simulink model "sim_all"  (R2020a)
settings: Solver=VariableStepAuto  StartTime=0.0  StopTime=2000  RelTol=1e-3
values from neighbouring files (symbols this model uses):
  a1 = rho * D^4 * alpha1    (= 0.000388302366464)    [data_current.m]
  a2 = -rho * D^3 * alpha2 * (1 - omega)    (= 0.0037030698432)    [data_current.m]
  alpha1 = 0.0113    [data_current.m]
  alpha2 = -0.0091    [data_current.m]
  cornerA = [43.781381 ... (first row only)    [missionC.m]
  cornerB = [43.780975 ... (first row only)    [missionC.m]
  cornerC = [43.780189 ... (first row only)    [missionC.m]
  cornerD = [43.780602 ... (first row only)    [missionC.m]
  ctrl_clockwise = false    [controller.m]
  ctrl_int_bound_or = 0.1    [controller.m]
  ctrl_int_bound_pos = 1    [controller.m]
  ctrl_k_or = 1    [controller.m]
  ctrl_k_pos = 1/3    (= 0.333333333333)    [controller.m]
  ctrl_Ki_vel = 100    [controller.m]
  ctrl_Kp_v_pos = 200    [controller.m]
  ctrl_Kp_vel = 200    [controller.m]
  ctrl_TAM = [  1     1           0           0               0       0;               0     0           1           1               0       0;               0     0           0           0               1       1;               0     0  -(ctrl_r+ctrl_dc)  ctrl_r+ctrl_dc    0       0;               0     0           0           0            -ctrl_r    ctrl_r;           -ctrl_r ctrl_r        0           0       ...(+19 chars)    [controller.m]
  ctrl_Ts = 0.1    [controller.m]
  ctrl_va_uncontrolled = 0.15    [controller.m]
  ctrl_vel_uncontrolled = 0.5    [controller.m]
  D = 0.076    [data_current.m]
  dead_zone_limit = 31.5    [data_current.m]
  depth = 5    [missionC.m]
  distanceFromWall = 8    [missionC.m]
  initInspectedSide = 2    [missionC.m]
  initPoint = [ 43.780796 ... (first row only)    [missionC.m]
  mod_A = pi*mod_R*mod_R    [model.m]
  mod_Cd_F = 0.45    [model.m]
  mod_Cd_M = 0.4    [model.m]
  mod_eta_init = [mod_xNorth; mod_yEast; -mod_zDown; 0; 0; 0]    [model.m]
  mod_g = 9.81    [model.m]
  mod_h0 = 0    [model.m]
  mod_Ixx = mod_Io(1,1)    [model.m]
  mod_Iyy = mod_Io(2,2)    [model.m]
  mod_Izz = mod_Io(3,3)    [model.m]
  mod_Kp_dot = 0    [model.m]
  mod_lat0 = 43.780189    [model.m]
  mod_lon0 = 11.282698    [model.m]
  mod_m = 100    [model.m]
  mod_Mq_dot = mod_Kp_dot    (= 0)    [model.m]
  mod_ni_init = [0; 0; 0; 0; 0; 0]    [model.m]
  mod_Nr_dot = mod_Kp_dot    (= 0)    [model.m]
  mod_p1 = [0; mod_R; 0]    [model.m]
  mod_p2 = [0; -mod_R; 0]    [model.m]
  mod_p3 = [0; 0; (mod_R + mod_z_cm)]    [model.m]
  mod_p4 = [0; 0; -(mod_R + mod_z_cm)]    [model.m]
  mod_p5 = [mod_R; 0; 0]    [model.m]
  mod_p6 = [-mod_R; 0; 0]    [model.m]
  mod_R = ((3*mod_Vol)/(4*pi))^(1/3)    [model.m]
  mod_Rm = (4*mod_R)/(3*pi)    [model.m]
  mod_t1 = [1; 0; 0]    [model.m]
  mod_t2 = [1; 0; 0]    [model.m]
  mod_t3 = [0; 1; 0]    [model.m]
  mod_t4 = [0; 1; 0]    [model.m]
  mod_t5 = [0; 0; 1]    [model.m]
  mod_t6 = [0; 0; 1]    [model.m]
  mod_W = mod_m*mod_g    (= 981)    [model.m]
  mod_Xu_dot = (2/3)*mod_rho_AUV*pi*(mod_R^3)    [model.m]
  mod_Yv_dot = mod_Xu_dot    [model.m]
  mod_z_cm = mod_r_cm(3)    [model.m]
  mod_Zw_dot = mod_Xu_dot    [model.m]
  n_max = 340    [data_current.m]
  nav_DT = 0.1    [navigation.m]
  nav_filter = -1    [data_analysis_simulation_total.m]    (also in navigation.m)
  nav_giro = 2    [navigation.m]
  nav_h0 = 0    [navigation.m]
  nav_lat0 = cornerC(1)    [navigation.m]
  nav_lon0 = cornerC(2)    [navigation.m]
  nav_plane_AB = coefficient_plane(nav_A,nav_B)    [navigation.m]
  nav_plane_BC = coefficient_plane(nav_B,nav_C)    [navigation.m]
  nav_plane_CD = coefficient_plane(nav_C,nav_D)    [navigation.m]
  nav_plane_DA = coefficient_plane(nav_D,nav_A)    [navigation.m]
  nav_resampling = 10000    [navigation.m]
  omega = 0.1    [data_current.m]
  relativeDirection = 30    [missionC.m]
  res_enable_n_eff = 1    [navigation.m]
  rho = 1030    [data_current.m]
  sens_distCM = 0.267    [sensors.m]
  sens_Sample_time_AHRS = 0.1    [sensors.m]
  sens_Sample_time_depth = 0.1    [sensors.m]
  sens_Sample_time_dvl = 0.2    [sensors.m]
  sens_Sample_time_GPS = 1    [sensors.m]
  sens_Sample_time_GYRO = 0.1    [sensors.m]
  sens_Sample_time_sonar = 0.5    [sensors.m]
  sens_threshold = 0.485    [sensors.m]
  sens_Variance_AHRS_pitch = (0.0087)^2    (= 7.569e-05)    [sensors.m]
  sens_Variance_AHRS_roll = (0.0087)^2    (= 7.569e-05)    [sensors.m]
  sens_Variance_AHRS_yaw = (0.0017)^2    (= 2.89e-06)    [sensors.m]
  sens_Variance_depth1 = (0.2)^2    (= 0.04)    [sensors.m]
  sens_Variance_depth2 = (0.4)^2    (= 0.16)    [sensors.m]
  sens_Variance_DVL = (speed*0.03)^2    [sensors.m]
  sens_Variance_GPS = 3    [sensors.m]
  sens_Variance_GYRO = 2.5133e-06    [sensors.m]
  sens_Variance_sonar = 0.05    [sensors.m]
  soglia_or = [0.1, 0.1, 0.1]    [mission.m]
  soglia_orp = 0.1    [mission.m]
  soglia_parete = 0.5    [mission.m]
  soglia_parete_frenata = 0.5    [mission.m]
  soglia_pos = [0.00001, 0.00001, 0.5]    [mission.m]
  soglia_SOS_collisione = 2    [mission.m]
  soglia_SOS_or = [0.25, 0.25, 0.25]    [mission.m]
  soglia_SOS_orp = 0.25    [mission.m]
  soglia_SOS_parete = 1    [mission.m]
  soglia_SOS_pos = [0.00005, 0.00005, 1]    [mission.m]
  soglia_SOS_pos_ris = 2    [mission.m]
  soglia_SOS_vel = 0.2    [mission.m]
  SOS = 0    [mission.m]
  speed = 0.4    [missionC.m]
  stato = 100    [mission.m]
  timer = 40*2    (= 80)    [mission.m]
  Ts_supervisor = 0.1    [mission.m]
undefined symbols (not defined in the file or in its folder): DiscIntNeverNeededParam, nav_A, nav_B, nav_C, nav_D
libraries: simulink x8, cstblocks x6, simulink_extras x1
(part 2 of 8)

== system sim_all/Controller_mk4_v3/C_vel ==
  note: CONSIDERAZIONI:
      | - il controllore è un PI costruito con sisotool
      | - il modello considerato è su un singolo asse con massa e damping
  err_vel : Inport
  enable : Inport  Port=2
  C_vel_X : simulink/Continuous/PID Controller  Controller=P  Form=Parallel  TimeDomain=Discrete-time  UseExternalTs=off  SampleTime=ctrl_Ts  IntegratorMethod=Forward Euler  FilterMethod=Forward Euler  ControllerParametersSource=internal  P=ctrl_Kp_vel  I=ctrl_Ki_vel  D=0  UseFilter=on  N=100  TunerSelectOption=Transfer Function Based (PID Tuner App)  InitialConditionSource=internal  InitialConditionForIntegrator=0  InitialConditionForFilter=0  DifferentiatorICPrevScaledInput=0  ExternalReset=rising  TrackingMode=off  Kt=1  LimitOutput=off  UpperSaturationLimit=inf  LowerSaturationLimit=-inf  LinearizeAsGain=on  AntiWindupMode=none  Kb=1  POutMin=[]  POutMax=[]  IOutMin=[]  IOutMax=[]  DOutMin=[]  DOutMax=[]  NOutMin=[]  NOutMax=[]  SumOutMin=[]  SumOutMax=[]  SaturationOutMin=[]  SaturationOutMax=[]  PParamMin=[]  PParamMax=[]  IParamMin=[]  IParamMax=[]  DParamMin=[]  DParamMax=[]  NParamMin=[]  NParamMax=[]  KbParamMin=[]  KbParamMax=[]  KtParamMin=[]  KtParamMax=[]  KbOutMin=[]  KbOutMax=[]  KtOutMin=[]  KtOutMax=[]  IntegratorOutMin=[]  IntegratorOutMax=[]  FilterOutMin=[]  FilterOutMax=[]  SumI1OutMin=[]  SumI1OutMax=[]  SumI2OutMin=[]  SumI2OutMax=[]  SumI3OutMin=[]  SumI3OutMax=[]  SumI4OutMin=[]  SumI4OutMax=[]  SumDOutMin=[]  SumDOutMax=[]  DifferentiatorOutMin=[]  DifferentiatorOutMax=[]  FilterDiffOutCoefMin=[]  FilterDiffOutCoefMax=[]  ReciprocalOutMin=[]  ReciprocalOutMax=[]  SumDenOutMin=[]  SumDenOutMax=[]  SumNumOutMin=[]  SumNumOutMax=[]  DivideOutMin=[]  DivideOutMax=[]  UdiffTsProdOutMin=[]  UdiffTsProdOutMax=[]  NTsProdOutMin=[]  NTsProdOutMax=[]  UintegralTsProdOutMin=[]  UintegralTsProdOutMax=[]  UngainTsProdOutMin=[]  UngainTsProdOutMax=[]  IntegratorContinuousStateAttributes=''  IntegratorStateMustResolveToSignalObject=off  IntegratorRTWStateStorageClass=Auto  FilterContinuousStateAttributes=''  FilterStateMustResolveToSignalObject=off  FilterRTWStateStorageClass=Auto  ParallelPVariant=InternalParameters  IdealPVariant=Disabled  IVariant=Disabled  DVariant=Disabled  IntegratorVariant=Disabled  SatVariant=Disabled  AWVariant=Disabled  PCopyVariant=Disabled  TRVariant=Disabled  FdbkBlocksVariant=Forward  IdealPFdbkVariant=Disabled  SatFdbkVariant=Disabled  DerivativeFilterVariant=Disabled  NVariant=Disabled  NCopyVariant=Disabled_SignalSpec  FilterICVariant=Disabled  IntegratorICVariant=Disabled  ExternalResetVariant=Disabled  TRSumVariant=Passthrough  SumFdbkVariant=Disabled  SumVariant=Passthrough_P  TsampFilterVariant=InternalTs  TsampNgainVariant=Passthrough  TsampIntegralVariant=Disabled_SignalSpec
  C_vel_Y : simulink/Continuous/PID Controller  Controller=P  Form=Parallel  TimeDomain=Discrete-time  UseExternalTs=off  SampleTime=ctrl_Ts  IntegratorMethod=Forward Euler  FilterMethod=Forward Euler  ControllerParametersSource=internal  P=ctrl_Kp_vel  I=ctrl_Ki_vel  D=0  UseFilter=on  N=100  TunerSelectOption=Transfer Function Based (PID Tuner App)  InitialConditionSource=internal  InitialConditionForIntegrator=0  InitialConditionForFilter=0  DifferentiatorICPrevScaledInput=0  ExternalReset=rising  TrackingMode=off  Kt=1  LimitOutput=off  UpperSaturationLimit=inf  LowerSaturationLimit=-inf  LinearizeAsGain=on  AntiWindupMode=none  Kb=1  POutMin=[]  POutMax=[]  IOutMin=[]  IOutMax=[]  DOutMin=[]  DOutMax=[]  NOutMin=[]  NOutMax=[]  SumOutMin=[]  SumOutMax=[]  SaturationOutMin=[]  SaturationOutMax=[]  PParamMin=[]  PParamMax=[]  IParamMin=[]  IParamMax=[]  DParamMin=[]  DParamMax=[]  NParamMin=[]  NParamMax=[]  KbParamMin=[]  KbParamMax=[]  KtParamMin=[]  KtParamMax=[]  KbOutMin=[]  KbOutMax=[]  KtOutMin=[]  KtOutMax=[]  IntegratorOutMin=[]  IntegratorOutMax=[]  FilterOutMin=[]  FilterOutMax=[]  SumI1OutMin=[]  SumI1OutMax=[]  SumI2OutMin=[]  SumI2OutMax=[]  SumI3OutMin=[]  SumI3OutMax=[]  SumI4OutMin=[]  SumI4OutMax=[]  SumDOutMin=[]  SumDOutMax=[]  DifferentiatorOutMin=[]  DifferentiatorOutMax=[]  FilterDiffOutCoefMin=[]  FilterDiffOutCoefMax=[]  ReciprocalOutMin=[]  ReciprocalOutMax=[]  SumDenOutMin=[]  SumDenOutMax=[]  SumNumOutMin=[]  SumNumOutMax=[]  DivideOutMin=[]  DivideOutMax=[]  UdiffTsProdOutMin=[]  UdiffTsProdOutMax=[]  NTsProdOutMin=[]  NTsProdOutMax=[]  UintegralTsProdOutMin=[]  UintegralTsProdOutMax=[]  UngainTsProdOutMin=[]  UngainTsProdOutMax=[]  IntegratorContinuousStateAttributes=''  IntegratorStateMustResolveToSignalObject=off  IntegratorRTWStateStorageClass=Auto  FilterContinuousStateAttributes=''  FilterStateMustResolveToSignalObject=off  FilterRTWStateStorageClass=Auto  ParallelPVariant=InternalParameters  IdealPVariant=Disabled  IVariant=Disabled  DVariant=Disabled  IntegratorVariant=Disabled  SatVariant=Disabled  AWVariant=Disabled  PCopyVariant=Disabled  TRVariant=Disabled  FdbkBlocksVariant=Forward  IdealPFdbkVariant=Disabled  SatFdbkVariant=Disabled  DerivativeFilterVariant=Disabled  NVariant=Disabled  NCopyVariant=Disabled_SignalSpec  FilterICVariant=Disabled  IntegratorICVariant=Disabled  ExternalResetVariant=Disabled  TRSumVariant=Passthrough  SumFdbkVariant=Disabled  SumVariant=Passthrough_P  TsampFilterVariant=InternalTs  TsampNgainVariant=Passthrough  TsampIntegralVariant=Disabled_SignalSpec
  C_vel_Z : simulink/Continuous/PID Controller  Controller=P  Form=Parallel  TimeDomain=Discrete-time  UseExternalTs=off  SampleTime=ctrl_Ts  IntegratorMethod=Forward Euler  FilterMethod=Forward Euler  ControllerParametersSource=internal  P=ctrl_Kp_vel  I=ctrl_Ki_vel  D=0  UseFilter=on  N=100  TunerSelectOption=Transfer Function Based (PID Tuner App)  InitialConditionSource=internal  InitialConditionForIntegrator=0  InitialConditionForFilter=0  DifferentiatorICPrevScaledInput=0  ExternalReset=rising  TrackingMode=off  Kt=1  LimitOutput=off  UpperSaturationLimit=inf  LowerSaturationLimit=-inf  LinearizeAsGain=on  AntiWindupMode=none  Kb=1  POutMin=[]  POutMax=[]  IOutMin=[]  IOutMax=[]  DOutMin=[]  DOutMax=[]  NOutMin=[]  NOutMax=[]  SumOutMin=[]  SumOutMax=[]  SaturationOutMin=[]  SaturationOutMax=[]  PParamMin=[]  PParamMax=[]  IParamMin=[]  IParamMax=[]  DParamMin=[]  DParamMax=[]  NParamMin=[]  NParamMax=[]  KbParamMin=[]  KbParamMax=[]  KtParamMin=[]  KtParamMax=[]  KbOutMin=[]  KbOutMax=[]  KtOutMin=[]  KtOutMax=[]  IntegratorOutMin=[]  IntegratorOutMax=[]  FilterOutMin=[]  FilterOutMax=[]  SumI1OutMin=[]  SumI1OutMax=[]  SumI2OutMin=[]  SumI2OutMax=[]  SumI3OutMin=[]  SumI3OutMax=[]  SumI4OutMin=[]  SumI4OutMax=[]  SumDOutMin=[]  SumDOutMax=[]  DifferentiatorOutMin=[]  DifferentiatorOutMax=[]  FilterDiffOutCoefMin=[]  FilterDiffOutCoefMax=[]  ReciprocalOutMin=[]  ReciprocalOutMax=[]  SumDenOutMin=[]  SumDenOutMax=[]  SumNumOutMin=[]  SumNumOutMax=[]  DivideOutMin=[]  DivideOutMax=[]  UdiffTsProdOutMin=[]  UdiffTsProdOutMax=[]  NTsProdOutMin=[]  NTsProdOutMax=[]  UintegralTsProdOutMin=[]  UintegralTsProdOutMax=[]  UngainTsProdOutMin=[]  UngainTsProdOutMax=[]  IntegratorContinuousStateAttributes=''  IntegratorStateMustResolveToSignalObject=off  IntegratorRTWStateStorageClass=Auto  FilterContinuousStateAttributes=''  FilterStateMustResolveToSignalObject=off  FilterRTWStateStorageClass=Auto  ParallelPVariant=InternalParameters  IdealPVariant=Disabled  IVariant=Disabled  DVariant=Disabled  IntegratorVariant=Disabled  SatVariant=Disabled  AWVariant=Disabled  PCopyVariant=Disabled  TRVariant=Disabled  FdbkBlocksVariant=Forward  IdealPFdbkVariant=Disabled  SatFdbkVariant=Disabled  DerivativeFilterVariant=Disabled  NVariant=Disabled  NCopyVariant=Disabled_SignalSpec  FilterICVariant=Disabled  IntegratorICVariant=Disabled  ExternalResetVariant=Disabled  TRSumVariant=Passthrough  SumFdbkVariant=Disabled  SumVariant=Passthrough_P  TsampFilterVariant=InternalTs  TsampNgainVariant=Passthrough  TsampIntegralVariant=Disabled_SignalSpec
  Constant3 : Constant  Value=0
  Constant4 : Constant  Value=0
  Constant5 : Constant  Value=0
  Demux1 : Demux  Outputs=3
  Mux2 : Mux  Inputs=6
  Sum5 : Sum  Inputs=++|
  Sum7 : Sum  Inputs=|++
  Sum8 : Sum  Inputs=++|
  Switch2 : Switch  Criteria=u2 ~= 0  Threshold=0.5
  Switch3 : Switch  Criteria=u2 ~= 0  Threshold=0.5
  abs_integrator : Subsystem
  tau_vel1 : Outport  VectorParamsAs1DForOutWhenUnconnected=off
  wires:
  C_vel_Y/1 -> Sum8/2
  C_vel_X/1 -> Sum7/1
  abs_integrator/1(int_vx) -> Sum7/2
  abs_integrator/3(int_vz) -> Sum5/1
  C_vel_Z/1 -> Sum5/2
  abs_integrator/2(int_vy) -> Sum8/1
  Switch2/1 -> Demux1/1
  err_vel/1 -> Switch2/1
  Constant3/1 -> Switch2/3
  Demux1/2 -> abs_integrator/2(err_vy), C_vel_Y/1
  Demux1/1 -> abs_integrator/1(err_vx), C_vel_X/1
  Demux1/3 -> C_vel_Z/1, abs_integrator/3(err_vz)
  Switch3/1 -> tau_vel1/1
  Mux2/1 -> Switch3/1
  Sum7/1 -> Mux2/1
  enable/1 -> abs_integrator/4(enabler), Switch3/2, Switch2/2
  Constant5/1 -> Switch3/3
  Sum5/1 -> Mux2/3
  Sum8/1 -> Mux2/2
  Constant4/1 -> Mux2/6, Mux2/5, Mux2/4

== system sim_all/Controller_mk4_v3/InputOr_Organizer ==
  prof_trig : Inport
  or_d : Inport  Port=2
  or_s : Inport  Port=3
  orp_ned : Inport  Port=4
  Switch4 : Switch  Criteria=u2 > Threshold  Threshold=0.5
  diff_or : MATLAB Function  TreatAsAtomicUnit=on
  err_or : Outport
  wires:
  diff_or/1(err_or) -> err_or/1
  Switch4/1 -> diff_or/1(or_d)
  prof_trig/1 -> Switch4/2
  or_d/1 -> Switch4/1
  orp_ned/1 -> Switch4/3
  or_s/1 -> diff_or/2(or_s)

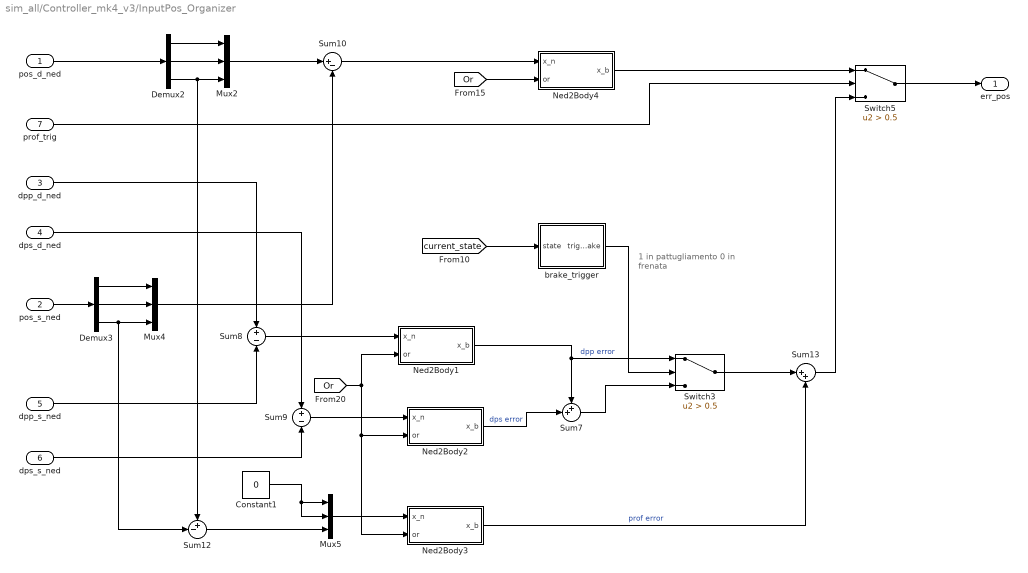
== system sim_all/Controller_mk4_v3/InputPos_Organizer ==
  note: 1 in pattugliamento
      | 0 in frenata
  pos_d_ned : Inport
  pos_s_ned : Inport  Port=2
  dpp_d_ned : Inport  Port=3
  dps_d_ned : Inport  Port=4
  dpp_s_ned : Inport  Port=5
  dps_s_ned : Inport  Port=6
  prof_trig : Inport  Port=7
  Constant1 : Constant  Value=0
  Demux2 : Demux  Outputs=3
  Demux3 : Demux  Outputs=3
  Mux2 : Mux  Inputs=3
  Mux4 : Mux  Inputs=3
  Mux5 : Mux  Inputs=3
  Ned2Body1 : MATLAB Function  TreatAsAtomicUnit=on
  Ned2Body2 : MATLAB Function  TreatAsAtomicUnit=on
  Ned2Body3 : MATLAB Function  TreatAsAtomicUnit=on
  Ned2Body4 : MATLAB Function  TreatAsAtomicUnit=on
  Sum10 : Sum  Inputs=|+-
  Sum12 : Sum  Inputs=+-|
  Sum13 : Sum  Inputs=|++
  Sum7 : Sum  Inputs=++|
  Sum8 : Sum  Inputs=+|-
  Sum9 : Sum  Inputs=+|-
  Switch3 : Switch  Criteria=u2 > Threshold  Threshold=0.5
  Switch5 : Switch  Criteria=u2 > Threshold  Threshold=0.5
  brake_trigger : MATLAB Function  TreatAsAtomicUnit=on
  err_pos : Outport
  wires:
  Sum13/1 -> Switch5/3
  Sum10/1 -> Ned2Body4/1(x_n)
  brake_trigger/1(trigg_brake) -> Switch3/2
  [Or] -> Ned2Body1/2(or), Ned2Body3/2(or), Ned2Body2/2(or)
  Switch3/1 -> Sum13/1
  Mux2/1 -> Sum10/1
  Switch5/1 -> err_pos/1
  Mux5/1 -> Ned2Body3/1(x_n)
  prof_trig/1 -> Switch5/2
  Ned2Body2/1(x_b) -> Sum7/2  "dps error"
  Ned2Body3/1(x_b) -> Sum13/2  "prof error"
  Sum8/1 -> Ned2Body1/1(x_n)
  dpp_d_ned/1 -> Sum8/1
  Demux2/3 -> Mux2/3, Sum12/1
  Mux4/1 -> Sum10/2
  Demux2/2 -> Mux2/2
  Ned2Body4/1(x_b) -> Switch5/1
  [Or] -> Ned2Body4/2(or)
  Demux3/3 -> Mux4/3, Sum12/2
  Ned2Body1/1(x_b) -> Switch3/1, Sum7/1  "dpp error"
  Demux2/1 -> Mux2/1
  Sum12/1 -> Mux5/3
  [current_state] -> brake_trigger/1(state)
  Sum9/1 -> Ned2Body2/1(x_n)
  Demux3/2 -> Mux4/2
  Constant1/1 -> Mux5/2, Mux5/1
  Sum7/1 -> Switch3/3
  Demux3/1 -> Mux4/1
  pos_s_ned/1 -> Demux3/1
  dps_s_ned/1 -> Sum9/2
  pos_d_ned/1 -> Demux2/1
  dps_d_ned/1 -> Sum9/1
  dpp_s_ned/1 -> Sum8/2

== system sim_all/Controller_mk4_v3/InputVel_Organizer ==
  vel_d_ned : Inport
  vel_s_body : Inport  Port=2
  Ned2Body4 : MATLAB Function  TreatAsAtomicUnit=on
  Sum11 : Sum  Inputs=|+-
  err_vel : Outport
  wires:
  Ned2Body4/1(x_b) -> Sum11/1
  vel_d_ned/1 -> Ned2Body4/1(x_n)
  Sum11/1 -> err_vel/1
  vel_s_body/1 -> Sum11/2
  [Or] -> Ned2Body4/2(or)

== system sim_all/Controller_mk4_v3/Mixer ==
  tau_pos : Inport
  tau_vel : Inport  Port=2
  tau_or : Inport  Port=3
  Mix : MATLAB Function  TreatAsAtomicUnit=on  SystemSampleTime=ctrl_Ts
  T2n : MATLAB Function  TreatAsAtomicUnit=on  SystemSampleTime=ctrl_Ts
  TAM1 : cstblocks/LTI System  sys=inv(ctrl_TAM)  IC=[]
  TAM2 : cstblocks/LTI System  sys=inv(ctrl_TAM)  IC=[]
  TAM3 : cstblocks/LTI System  sys=inv(ctrl_TAM)  IC=[]
  n : Outport  VectorParamsAs1DForOutWhenUnconnected=off
  wires:
  Mix/1(T) -> T2n/1(T)
  TAM3/1 -> Mix/3(To)
  TAM2/1 -> Mix/2(Tv)
  TAM1/1 -> Mix/1(Tp)
  tau_pos/1 -> TAM1/1
  tau_vel/1 -> TAM2/1
  T2n/1(n) -> n/1
  tau_or/1 -> TAM3/1

== system sim_all/Controller_mk4_v3/signal_to_NED ==
  Vel_d : Inport
  Dpp_d : Inport  Port=2
  Dps_d : Inport  Port=3
  Orp_d : Inport  Port=4
  Dpp_s : Inport  Port=5
  Dps_s : Inport  Port=6
  Signal_d->NED : Subsystem
  Signal_s->NED : Subsystem
  prof_trigger : MATLAB Function  TreatAsAtomicUnit=on
  Dpp_d_ned : Outport
  Dps_d_ned : Outport  Port=2
  Dpp_s_ned : Outport  Port=3
  Dps_s_ned : Outport  Port=4
  trigg_prof : Outport  Port=5
  Vel_d_ned : Outport  Port=6
  Orp_d_ned : Outport  Port=7
  wires:
  Dps_s/1 -> Signal_s->NED/2(Dps_s)
  [current_state] -> prof_trigger/1(state)
  [parete_attuale] -> Signal_d->NED/5(Wall)
  [parete_attuale] -> Signal_s->NED/3(Wall)
  Signal_d->NED/4(Orp_d_ned) -> Orp_d_ned/1
  Vel_d/1 -> Signal_d->NED/1(Vel_d)
  Dpp_d/1 -> Signal_d->NED/2(Dpp_d)
  Signal_d->NED/3(Dps_d_ned) -> Dps_d_ned/1
  Signal_d->NED/2(Dpp_d_ned) -> Dpp_d_ned/1
  Orp_d/1 -> Signal_d->NED/4(Orp_d)
  Dps_d/1 -> Signal_d->NED/3(Dps_d)
  Signal_s->NED/2(Dps_s_ned) -> Dps_s_ned/1
  Dpp_s/1 -> Signal_s->NED/1(Dpp_s)
  prof_trigger/1(trigg_prof) -> trigg_prof/1
  Signal_s->NED/1(Dpp_s_ned) -> Dpp_s_ned/1
  Signal_d->NED/1(Vel_d_ned) -> Vel_d_ned/1

== system sim_all/EKF/Calcolo distaza pareti ==
  orient : Inport
  pos_es : Inport  Port=2
  Calcolo distanza dalle pareti : MATLAB Function  TreatAsAtomicUnit=on
  Calcolo orientazione dalla parete : MATLAB Function  TreatAsAtomicUnit=on
  dpp : Outport
  dps : Outport  Port=2
  orient_parete : Outport  Port=3
  wires:
  pos_es/1 -> Calcolo distanza dalle pareti/1(pos_es), Calcolo orientazione dalla parete/1(pos_es)
  Calcolo distanza dalle pareti/2(dps) -> dps/1
  Calcolo orientazione dalla parete/1(orient_parete) -> orient_parete/1
  orient/1 -> Calcolo orientazione dalla parete/3(orient)
  Calcolo distanza dalle pareti/1(dpp) -> dpp/1
  [parete_attuale] -> Calcolo distanza dalle pareti/2(parete_attuale), Calcolo orientazione dalla parete/2(parete_attuale)

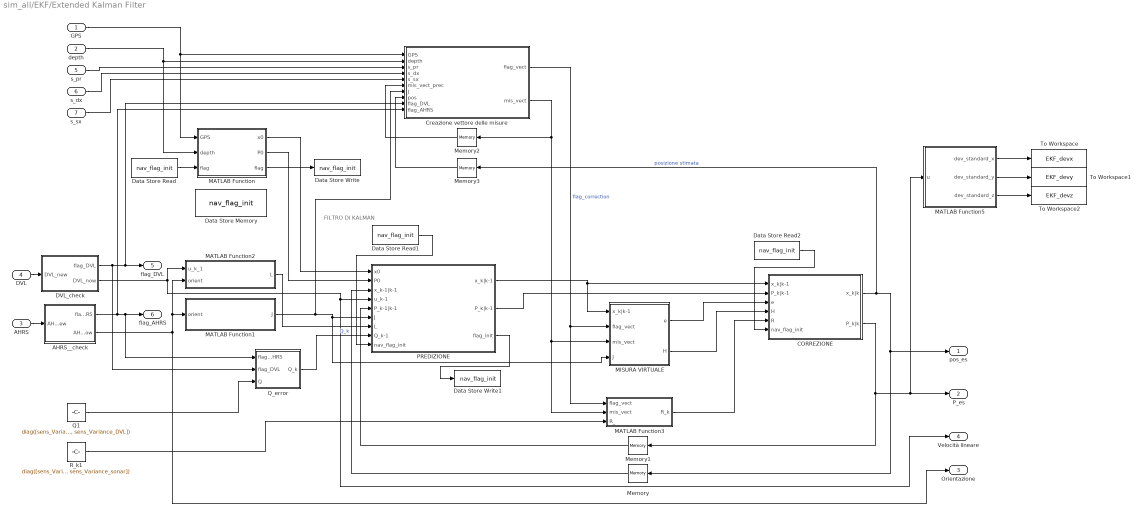
== system sim_all/EKF/Extended Kalman Filter ==
  note: FILTRO DI KALMAN
  GPS : Inport
  depth : Inport  Port=2
  AHRS : Inport  Port=3
  DVL : Inport  Port=4
  s_pr : Inport  Port=5
  s_dx : Inport  Port=6
  s_sx : Inport  Port=7
  AHRS__check : Subsystem
  CORREZIONE : Subsystem
  Creazione vettore delle misure : MATLAB Function  TreatAsAtomicUnit=on  SystemSampleTime=nav_DT
  DVL_check : Subsystem
  Data Store Memory : DataStoreMemory  DataStoreName=nav_flag_init  ShowAdditionalParam=off
  Data Store Read : DataStoreRead  DataStoreName=nav_flag_init  DataStoreElements=nav_flag_init
  Data Store Read1 : DataStoreRead  DataStoreName=nav_flag_init  DataStoreElements=nav_flag_init
  Data Store Read2 : DataStoreRead  DataStoreName=nav_flag_init  DataStoreElements=nav_flag_init
  Data Store Write : DataStoreWrite  DataStoreName=nav_flag_init  DataStoreElements=nav_flag_init
  Data Store Write1 : DataStoreWrite  DataStoreName=nav_flag_init  DataStoreElements=nav_flag_init
  MATLAB Function : MATLAB Function  TreatAsAtomicUnit=on
  MATLAB Function1 : MATLAB Function  TreatAsAtomicUnit=on
  MATLAB Function2 : MATLAB Function  TreatAsAtomicUnit=on
  MATLAB Function3 : MATLAB Function  TreatAsAtomicUnit=on  SystemSampleTime=nav_DT
  MATLAB Function5 : MATLAB Function  TreatAsAtomicUnit=on
  MISURA VIRTUALE : Subsystem
  Memory{,1..3} (4 alike) : Memory
  PREDIZIONE : Subsystem
  Q1 : Constant  Value=diag([sens_Variance_AHRS_roll, sens_Variance_AHRS_pitch, sens_Variance_AHRS_yaw, sens_Variance_DVL, sens_Variance_DVL, sens_Variance_DVL])  VectorParams1D=off
  Q_error : Subsystem
  R_k1 : Constant  Value=diag([sens_Variance_GPS, sens_Variance_GPS, sens_Variance_depth1, sens_Variance_sonar, sens_Variance_sonar, sens_Variance_sonar])  VectorParams1D=off
  To Workspace : ToWorkspace  VariableName=EKF_devx  SaveFormat=Timeseries  SampleTime=0.1
      settings: Decimation=10
  To Workspace1 : ToWorkspace  VariableName=EKF_devy  SaveFormat=Timeseries  SampleTime=0.1
      settings: Decimation=10
  To Workspace2 : ToWorkspace  VariableName=EKF_devz  SaveFormat=Timeseries  SampleTime=0.1
      settings: Decimation=10
  pos_es : Outport
  P_es : Outport  Port=2
  Orientazione : Outport  Port=3
  Velocità lineare : Outport  Port=4
  flag_DVL : Outport  Port=5
  flag_AHRS : Outport  Port=6
  wires:
  PREDIZIONE/1(x_k|k-1) -> MISURA VIRTUALE/1(x_k|k-1), CORREZIONE/1(x_k|k-1)
  PREDIZIONE/2(P_k|k-1) -> CORREZIONE/2(P_k|k-1)
  Memory/1 -> PREDIZIONE/3(x_k-1|k-1)
  CORREZIONE/2(P_k|k) -> Memory1/1, P_es/1, MATLAB Function5/1(u)
  Memory1/1 -> PREDIZIONE/5(P_k-1|k-1)
  MISURA VIRTUALE/2(H) -> CORREZIONE/4(H)
  MISURA VIRTUALE/1(e) -> CORREZIONE/3(e)
  GPS/1 -> MATLAB Function/1(GPS), Creazione vettore delle misure/1(GPS)
  depth/1 -> MATLAB Function/2(depth), Creazione vettore delle misure/2(depth)
  s_pr/1 -> Creazione vettore delle misure/3(s_pr)
  Creazione vettore delle misure/2(mis_vect) -> MATLAB Function3/2(mis_vect), MISURA VIRTUALE/3(mis_vect), Memory2/1
  Memory2/1 -> Creazione vettore delle misure/6(mis_vect_prec)
  Creazione vettore delle misure/1(flag_vect) -> MATLAB Function3/1(flag_vect), MISURA VIRTUALE/2(flag_vect)  "flag_correction"
  s_dx/1 -> Creazione vettore delle misure/4(s_dx)
  s_sx/1 -> Creazione vettore delle misure/5(s_sx)
  MATLAB Function/2(P0) -> PREDIZIONE/2(P0)
  MATLAB Function/1(x0) -> PREDIZIONE/1(x0)
  MATLAB Function1/1(J) -> Creazione vettore delle misure/7(J), MISURA VIRTUALE/4(J), PREDIZIONE/6(J)
  MATLAB Function2/1(L) -> PREDIZIONE/7(L)
  Data Store Read/1 -> MATLAB Function/3("flag ")
  MATLAB Function/3(flag) -> Data Store Write/1
  Data Store Read1/1 -> PREDIZIONE/9(nav_flag_init)
  Data Store Read2/1 -> CORREZIONE/6(nav_flag_init)
  PREDIZIONE/3(flag_init) -> Data Store Write1/1
  R_k1/1 -> MATLAB Function3/3(R_)
  MATLAB Function3/1(R_k) -> CORREZIONE/5(R)
  CORREZIONE/1(x_k|k) -> pos_es/1, Memory/1, Memory3/1  "posizione stimata"
  Memory3/1 -> Creazione vettore delle misure/8(pos)
  AHRS__check/2(AHRS_now) -> Orientazione/1, MATLAB Function2/2(orient), MATLAB Function1/1(orient)
  DVL_check/2(DVL_now) -> Velocità lineare/1, PREDIZIONE/4(u_k-1), MATLAB Function2/1(u_k_1)
  DVL/1 -> DVL_check/1(DVL_new)
  AHRS/1 -> AHRS__check/1(AHRS_new)
  DVL_check/1(flag_DVL) -> flag_DVL/1, Creazione vettore delle misure/9(flag_DVL), Q_error/2(flag_DVL)
  AHRS__check/1(flag_AHRS) -> flag_AHRS/1, Q_error/1(flag_AHRS), Creazione vettore delle misure/10(flag_AHRS)
  Q1/1 -> Q_error/3(Q)
  Q_error/1(Q_k) -> PREDIZIONE/8(Q_k-1)  "Q_k"
  MATLAB Function5/1(dev_standard_x) -> To Workspace/1
  MATLAB Function5/2(dev_standard_y) -> To Workspace1/1
  MATLAB Function5/3(dev_standard_z) -> To Workspace2/1

== system sim_all/EKF/Filtro AHRS ==
  AHRS : Inport
  Filtro 1 : DiscreteFir  Coefficients=[0.2 0.2 0.2 0.1 0.1 0.1 0.1]  SampleTime=0.1
  Orientazione : Outport
  wires:
  AHRS/1 -> Filtro 1/1
  Filtro 1/1 -> Orientazione/1

== system sim_all/EKF/Filtro DVL ==
  DVL : Inport
  Demux : Demux  Outputs=3
  Filtro 2 : DiscreteFir  Coefficients=[0.3 0.3 0.2 0.2]  SampleTime=0.1
  Filtro 3 : DiscreteFir  Coefficients=[0.3 0.3 0.2 0.2]  SampleTime=0.1
  Mux : Mux  Inputs=3
  Velocità lineare : Outport
  wires:
  Filtro 2/1 -> Mux/1
  Demux/3 -> Mux/3
  DVL/1 -> Demux/1
  Filtro 3/1 -> Mux/2
  Mux/1 -> Velocità lineare/1  "DVL"
  Demux/1 -> Filtro 2/1
  Demux/2 -> Filtro 3/1

== system sim_all/EKF/Filtro Gyro ==
  Gyro : Inport
  Filtro 1 : DiscreteFir  Coefficients=[0.9 0.05 0.05]  SampleTime=0.1
  Velocità Angolare : Outport
  wires:
  Gyro/1 -> Filtro 1/1
  Filtro 1/1 -> Velocità Angolare/1

== system sim_all/EKF/Gyro_check ==
  Gyro_new : Inport
  MATLAB Function4 : MATLAB Function  TreatAsAtomicUnit=on
  Memory4 : Memory
  flag_Gyro : Outport
  Gyro_now : Outport  Port=2
  wires:
  Gyro_new/1 -> MATLAB Function4/1(gyro_new)
  Memory4/1 -> MATLAB Function4/2(gyro_old)
  MATLAB Function4/1(flag_gyro) -> flag_Gyro/1
  MATLAB Function4/2(gyro_now) -> Memory4/1, Gyro_now/1

== system sim_all/EKF/SOS_flag_generator ==
  P_es : Inport
  AHRS : Inport  Port=2
  DVL : Inport  Port=3
  Gyro : Inport  Port=4
  MATLAB Function : MATLAB Function  TreatAsAtomicUnit=on  SystemSampleTime=nav_DT
  Memory : Memory
  nav_SOS : Outport
  tag scope: nav_contatore=global
  wires:
  MATLAB Function/1(SOS) -> nav_SOS/1
  AHRS/1 -> MATLAB Function/3(AHRS)
  DVL/1 -> MATLAB Function/2(DVL)
  P_es/1 -> MATLAB Function/1(P_es)
  [nav_contatore] -> Memory/1
  MATLAB Function/2(contatore) -> [nav_contatore]
  Gyro/1 -> MATLAB Function/4(gyro)
  Memory/1 -> MATLAB Function/5("contatore ")

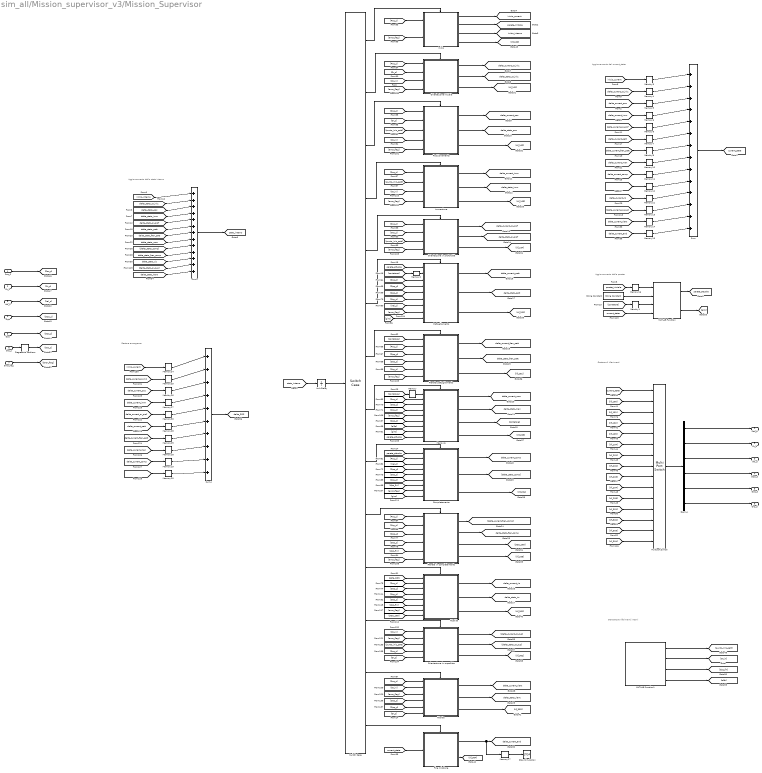
== system sim_all/Mission_supervisor_v3/Mission_Supervisor ==
  note: Gestore emergenza
  note: Generatore riferimenti interni
  note: Aggiornamento dello stato interno
  note: Aggiornamento del current_state
  note: Aggiornamento della parete
  note: Gestore di riferimenti
  Pos_S : Inport
  Or_S : Inport  Port=2
  Vel_S : Inport  Port=3
  Dpp : Inport  Port=4
  Dps : Inport  Port=5
  Orp_s : Inport  Port=6
  error_flag : Inport  Port=7
  Completamento : Subsystem  TreatAsAtomicUnit=on
  Degrees to Radians : simulink_extras/Transformations/Degrees to Radians
  Demux : Demux  Outputs=[3,3,1,1,1,1]
  Fine missione : Subsystem  TreatAsAtomicUnit=on
  Frenata in completamento : Subsystem  TreatAsAtomicUnit=on
  Frenata pattugliamento : Subsystem  TreatAsAtomicUnit=on
  Immersione : Subsystem  TreatAsAtomicUnit=on
  Inizio : Subsystem  TreatAsAtomicUnit=on
  MATLAB Function : MATLAB Function  TreatAsAtomicUnit=on
  MATLAB Function1 : MATLAB Function  TreatAsAtomicUnit=on
  Manovra : Subsystem  TreatAsAtomicUnit=on
  Memory{,1..2,4..15,17..21,25..30} (26 alike) : Memory
  Memory16 : Memory  InitialCondition=initInspectedSide
  Memory24 : Memory  InitialCondition=100
  Memory3 : Memory  InitialCondition=100
  Multiport Switch : MultiPortSwitch  DataPortOrder=Specify indices  Inputs=2  DataPortIndices={100,101,102,103,104,201,202,203,204,205,301,302,303,304}
  Orientazione Iniziale : Subsystem  TreatAsAtomicUnit=on
  Orientazione in profondità : Subsystem  TreatAsAtomicUnit=on
  Orientazione in superficie : Subsystem  TreatAsAtomicUnit=on
  Pattugliamento : Subsystem  TreatAsAtomicUnit=on
  Posizionamento : Subsystem  TreatAsAtomicUnit=on
  Rientro : Subsystem  TreatAsAtomicUnit=on
  Risalita : Subsystem  TreatAsAtomicUnit=on
  Stop Simulation : Stop
  String Constant : StringConstant  String=inspectionDirection
  Sum : Sum  Inputs=|++++++++++++++
  Sum1 : Sum  Inputs=|+++++++++++++
  Sum4 : Sum  Inputs=|++++++++++
  Switch Case : SwitchCase  CaseConditions={100,101,102,103,104,201,202,203,204,205,301,302,303,304}  ShowDefaultCase=off
  Unit Delay : UnitDelay  InitialCondition=stato  SampleTime=Ts_supervisor  HasFrameUpgradeWarning=on
  Pos_d : Outport
  Or_d : Outport  Port=2
  Vel_d : Outport  Port=3
  Dpp_d : Outport  Port=4
  Dps_d : Outport  Port=5
  Orp_d : Outport  Port=6
  tag scope: current_state=global, delta_SOS=global, delta_current_comp=global, delta_current_end=global, delta_current_fren_patt=global, delta_current_imm=global, delta_current_man=global, delta_current_or_iniz=global, delta_current_or_prof=global, delta_current_patt=global, delta_current_pos=global, delta_current_rient=global, delta_current_ris=global, delta_stato_fren_comp=global, delta_stato_fren_patt=global, delta_stato_imm=global, delta_stato_man=global, delta_stato_or_iniz=global, delta_stato_or_prof=global, delta_stato_patt=global, delta_stato_pos=global, delta_stato_rient=global, delta_stato_ris=global, inizio_current=global, inizio_interno=global, parete_attuale=global, parete_iniziale=global, stato_interno=global
  wires:
  [delta_stato_fren_comp] -> Sum1/10
  [delta_SOS] -> Risalita/1(delta_SOS)
  [delta_current_patt] -> Memory7/1
  [delta_current_pos] -> Memory5/1
  Immersione/1(delta_current_immers) -> [delta_current_imm]
  Posizionamento/3(Outport) -> [rif_102]
  Rientro/2(delta_stato_rient) -> [delta_stato_rient]
  [delta_stato_or_iniz] -> Sum1/2
  [inizio_interno] -> Sum1/1
  Memory6/1 -> Sum/4
  Orientazione Iniziale/1(delta_current_or_iniz) -> [delta_current_or_iniz]
  [delta_current_end] -> Memory15/1
  Pattugliamento/1(delta_current_patt) -> [delta_current_patt]
  Memory15/1 -> Sum/14
  Orientazione in profondità/2(delta_stato_or_prof) -> [delta_stato_or_prof]
  Memory12/1 -> Sum/10
  Memory8/1 -> Sum/7
  Completamento/3(Outport) -> [rif_204]
  Pattugliamento/2(delta_stato_patt) -> [delta_stato_patt]
  [delta_stato_man] -> Sum1/8
  Frenata in completamento/1(delta_current_fren_comp) -> [delta_current_fren_comp]
  Frenata pattugliamento/1(delta_current_fren_patt) -> [delta_current_fren_patt]
  Sum/1 -> [current_state]
  Inizio/1(current_state) -> [inizio_current]
  Memory4/1 -> Sum/2
  Posizionamento/2(delta_stato_posiz) -> [delta_stato_pos]
  [delta_stato_pos] -> Sum1/3
  Completamento/2(delta_stato_comp) -> [delta_stato_comp]
  [contatore] -> Memory2/1
  Memory17/1 -> Stop Simulation/1
  [delta_stato_imm] -> Sum1/4
  [delta_current_imm] -> Memory6/1
  [stato_interno] -> Unit Delay/1
  Sum1/1 -> [stato_interno]
  Inizio/2(parete_attuale) -> [parete_iniziale]
  [delta_stato_comp] -> Sum1/9
  [delta_stato_patt] -> Sum1/6
  Risalita/2(delta_stato_ris) -> [delta_stato_ris]
  [delta_current_fren_patt] -> Memory8/1
  [delta_current_or_prof] -> Memory9/1
  Rientro/1(delta_current_rient) -> [delta_current_rient]
  [current_state] -> Fine missione/1(current_state)
  Unit Delay/1 -> Switch Case/1
  [parete_attuale] -> Pattugliamento/1(parete)
  Memory7/1 -> Sum/6
  Orientazione in profondità/1(delta_current_or_prof) -> [delta_current_or_prof]
  Frenata in completamento/2(delta_stato_fren_comp) -> [delta_stato_fren_comp]
  [contatore] -> Frenata pattugliamento/1(contatore)
  Manovra/1(delta_current_man) -> [delta_current_man]
  [delta_current_fren_comp] -> Memory12/1
  Fine missione/1(delta_current_end) -> [delta_current_end], Memory17/1
  [inizio_current] -> Memory3/1
  [parete_attuale] -> Completamento/1(parete)
  Memory3/1 -> Sum/1
  Risalita/1(delta_current_ris) -> [delta_current_ris]
  [delta_stato_or_prof] -> Sum1/5
  Memory2/1 -> Pattugliamento/2(contatore)
  Memory11/1 -> Sum/9
  Posizionamento/1(delta_current_posiz) -> [delta_current_pos]
  Rientro/3(Outport) -> [rif_303]
  Inizio/3(delta_stato) -> [inizio_interno]
  [delta_current_comp] -> Memory11/1
  [delta_stato_fren_patt] -> Sum1/7
  [delta_stato_ris] -> Sum1/11
  Orientazione in profondità/3(Outport) -> [rif_104]
  Frenata pattugliamento/3(Outport) -> [rif_202]
  Orientazione Iniziale/2(delta_stato_or_iniz) -> [delta_stato_or_iniz]
  Fine missione/2(Outport) -> [rif_304]
  Memory10/1 -> Sum/8
  [delta_current_man] -> Memory10/1
  Immersione/2(delta_stato_immers) -> [delta_stato_imm]
  Manovra/2(delta_stato_man) -> [delta_stato_man]
  Orientazione Iniziale/3(Outport) -> [rif_101]
  [delta_current_or_iniz] -> Memory4/1
  Pattugliamento/3(Outport) -> [rif_201]
  Frenata pattugliamento/2(delta_stato_fren_patt) -> [delta_stato_fren_patt]
  Memory9/1 -> Sum/5
  Memory14/1 -> Sum/13
  Inizio/4(Outport) -> [rif_100]
  Risalita/3(Outport) -> [rif_301]
  Immersione/3(Outport) -> [rif_103]
  Memory5/1 -> Sum/3
  [Pos_s] -> Inizio/1(Pos_s)
  [Pos_s] -> Orientazione Iniziale/1(Pos_s)
  [Pos_s] -> Posizionamento/1(Pos_s)
  [Pos_s] -> Immersione/1(Pos_s)
  [Pos_s] -> Frenata pattugliamento/2(Pos_s)
  [Dpp_s] -> Frenata pattugliamento/3(Dpp_s)
  [Dps_s] -> Frenata pattugliamento/4(Dps_s)
  [Pos_s] -> Pattugliamento/3(Pos_s)
  [Dpp_s] -> Pattugliamento/4(Dpp_s)
  [Dps_s] -> Pattugliamento/5(Dps_s)
  [Orp_s] -> Pattugliamento/6(Orp_s)
  [Vel_s] -> Pattugliamento/7(Vel_s)
  [Orp_s] -> Frenata pattugliamento/5(Orp_s)
  [Dpp_s] -> Manovra/3(Dpp_s)
  [Orp_s] -> Manovra/4(Orp_s)
  [Pos_s] -> Manovra/2(Pos_s)
  [Pos_s] -> Completamento/2(Pos_s)
  [Vel_s] -> Completamento/3(Vel_s)
  [Dpp_s] -> Completamento/4(Dpp_s)
  [Dps_s] -> Completamento/5(Dps_s)
  [Orp_s] -> Completamento/6(Orp_s)
  [Pos_s] -> Frenata in completamento/1(Pos_s)
  [Orp_s] -> Frenata in completamento/2(Orp_s)
  [Dpp_s] -> Frenata in completamento/3(Dpp_s)
  [Dps_s] -> Frenata in completamento/4(Dps_s)
  [Pos_s] -> Risalita/2(Pos_s)
  [Dpp_s] -> Risalita/3(Dpp_s)
  [Pos_s] -> Rientro/1(Pos_s)
  Demux/2 -> Or_d/1
  [rif_202] -> Multiport Switch/8
  [current_state] -> Multiport Switch/1
  Demux/6 -> Orp_d/1
  Demux/3 -> Vel_d/1
  Multiport Switch/1 -> Demux/1
  [rif_301] -> Multiport Switch/12
  Demux/4 -> Dpp_d/1
  [rif_102] -> Multiport Switch/4
  [rif_203] -> Multiport Switch/9
  Demux/5 -> Dps_d/1
  Demux/1 -> Pos_d/1
  [rif_302] -> Multiport Switch/13
  [rif_201] -> Multiport Switch/7
  [rif_104] -> Multiport Switch/6
  [rif_205] -> Multiport Switch/11
  [rif_204] -> Multiport Switch/10
  [rif_101] -> Multiport Switch/3
  [rif_303] -> Multiport Switch/14
  [rif_103] -> Multiport Switch/5
  Completamento/1(delta_current_comp) -> [delta_current_comp]
  [Pos_s] -> Orientazione in profondità/1(Pos_s)
  [Orp_s] -> Orientazione in profondità/2(Orp_s)
  [rif_100] -> Multiport Switch/2
  [Or_s] -> Orientazione Iniziale/2(Or_s)
  [Or_in] -> Orientazione Iniziale/3(Or_in)
  [Or_in] -> Posizionamento/4(Or_in)
  [punto_iniz_patt] -> Posizionamento/3(punto iniziale)
  [dps_fin] -> Frenata in completamento/5(dps_fin)
  [punto_iniz_patt] -> Immersione/2(punto_iniz_patt)
  [punto_iniz_patt] -> Orientazione in profondità/3(Punto_iniz_patt)
  [Or_s] -> Posizionamento/2(Or_s)
  [dps_fin] -> Completamento/7(Dps_fin)
  error_flag/1 -> [error_flag]
  [error_flag] -> Frenata in completamento/6(error_flag)
  [error_flag] -> Completamento/8(error_flag)
  [error_flag] -> Manovra/5(error_flag)
  [error_flag] -> Frenata pattugliamento/6(error_flag)
  [error_flag] -> Pattugliamento/8(error_flag)
  [error_flag] -> Orientazione in profondità/4(error_flag)
  [error_flag] -> Immersione/4(error_flag)
  [error_flag] -> Posizionamento/5(error_flag)
  [error_flag] -> Orientazione Iniziale/4(error_flag)
  [error_flag] -> Inizio/2(error_flag)
  MATLAB Function1/3(dps_fin) -> [dps_fin]
  MATLAB Function1/2(Or_in) -> [Or_in]
  MATLAB Function1/1(punto_iniz_patt) -> [punto_iniz_patt]
  [Or_in] -> Immersione/3(Or_in)
  [Or_in] -> Rientro/2(Or_in)
  Memory25/1 -> Sum4/2
  Sum4/1 -> [delta_SOS]
  Memory27/1 -> Sum4/4
  Memory20/1 -> Sum4/10
  [delta_current_fren_comp] -> Memory20/1
  Memory26/1 -> Sum4/3
  Memory28/1 -> Sum4/6
  [delta_current_comp] -> Memory19/1
  Memory18/1 -> Sum4/8
  [delta_current_or_prof] -> Memory30/1
  Memory30/1 -> Sum4/5
  [delta_current_or_iniz] -> Memory25/1
  [delta_current_man] -> Memory18/1
  [delta_current_fren_patt] -> Memory29/1
  [delta_current_patt] -> Memory28/1
  [inizio_current] -> Memory24/1
  [delta_current_pos] -> Memory26/1
  [delta_current_imm] -> Memory27/1
  Memory24/1 -> Sum4/1
  Memory29/1 -> Sum4/7
  Memory19/1 -> Sum4/9
  [contatore] -> Memory1/1
  [parete_iniziale] -> Memory16/1
  [current_state] -> MATLAB Function/4(current_state)
  Memory1/1 -> MATLAB Function/3(contatore)
  String Constant/1 -> MATLAB Function/2(verso)
  Memory16/1 -> MATLAB Function/1(parete_iniziale)
  MATLAB Function/1(parete) -> [parete_attuale]
  [contatore] -> Memory/1
  Memory/1 -> Manovra/1(contatore)
  [Dps_s] -> Risalita/5(Dps_s)
  [Orp_s] -> Risalita/4(Orp_s)
  [dps_fin] -> Risalita/6(Dps_fin)
  Switch Case/1 -> Inizio/Action
  Switch Case/3 -> Posizionamento/Action
  Switch Case/2 -> Orientazione Iniziale/Action
  Switch Case/4 -> Immersione/Action
  Switch Case/5 -> Orientazione in profondità/Action
  Switch Case/6 -> Pattugliamento/Action
  Switch Case/7 -> Frenata pattugliamento/Action
  Switch Case/8 -> Manovra/Action
  Switch Case/9 -> Completamento/Action
  Switch Case/10 -> Frenata in completamento/Action
  Switch Case/11 -> Risalita/Action
  Switch Case/12 -> Orientazione in superficie/Action
  Switch Case/13 -> Rientro/Action
  Switch Case/14 -> Fine missione/Action
  Orientazione in superficie/1(delta_current_or_sup) -> [delta_current_or_sup]
  Orientazione in superficie/2(delta_stato_or_sup) -> [delta_stato_or_sup]
  Orientazione in superficie/3(Outport) -> [rif_302]
  [rif_304] -> Multiport Switch/15
  [error_flag] -> Risalita/7(error_flag)
  Memory13/1 -> Sum/12
  Memory21/1 -> Sum/11
  [delta_stato_or_sup] -> Sum1/12
  [delta_stato_rient] -> Sum1/13
  [delta_current_rient] -> Memory14/1
  [delta_current_or_sup] -> Memory13/1
  [delta_current_ris] -> Memory21/1
  [error_flag] -> Rientro/3(error_flag)
  [error_flag] -> Orientazione in superficie/2(error_flag)
  [Or_in] -> Orientazione in superficie/1(Or_in)
  [punto_iniz_patt] -> Orientazione in superficie/3(punto_iniz_patt)
  [Or_s] -> Orientazione in superficie/5(Or_s)
  [Pos_s] -> Orientazione in superficie/4(Pos_s)
  [Dps_s] -> Rientro/4(Dps_s)
  [Dpp_s] -> Rientro/5(Dpp_s)
  [Dps_s] -> Manovra/6(Dps_s)
  MATLAB Function/2(giro) -> [giro]
  [giro] -> Pattugliamento/9(giro)
  [giro] -> Completamento/9(giro)
  [SOS_205] -> Risalita/8(SOS_205)
  Pos_S/1 -> [Pos_s]
  Or_S/1 -> [Or_s]
  Vel_S/1 -> [Vel_s]
  Dpp/1 -> [Dpp_s]
  Dps/1 -> [Dps_s]
  Orp_s/1 -> Degrees to Radians/1
  Degrees to Radians/1 -> [Orp_s]
  Manovra/4("  ") -> [rif_203]
  Manovra/3(contatore_out) -> [contatore]
  Frenata in completamento/3(SOS_205) -> [SOS_205]
  Frenata in completamento/4(" ") -> [rif_205]
  [Or_s] -> Rientro/6(Or_s)
  MATLAB Function1/4(alfa) -> [alfa]
  [alfa] -> Manovra/7(alfa)
  [giro] -> Manovra/8(giro)
  [parete_attuale] -> Manovra/9(parete_attuale)

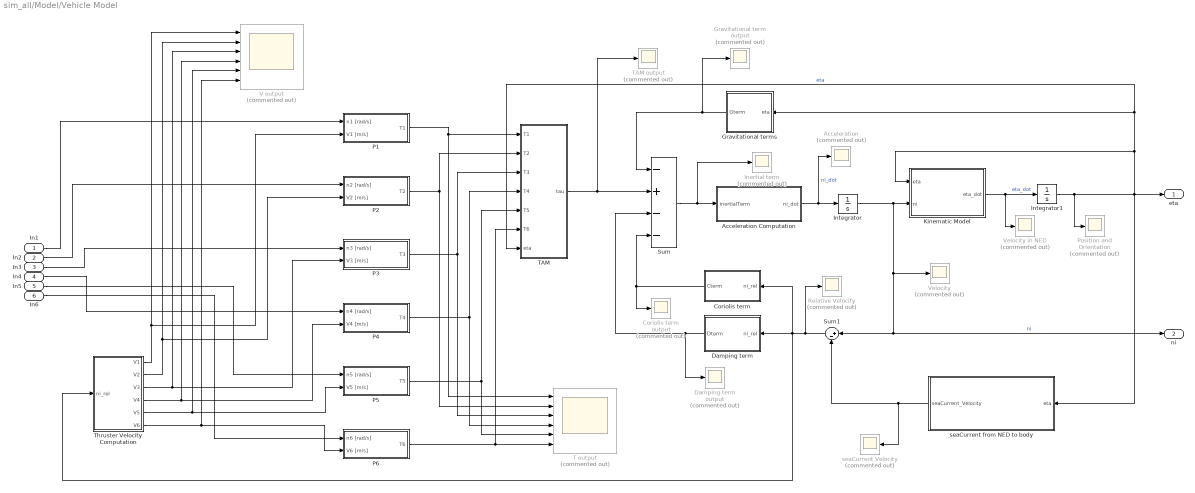
== system sim_all/Model/Vehicle Model ==
  In1 : Inport
  In2 : Inport  Port=2
  In3 : Inport  Port=3
  In4 : Inport  Port=4
  In5 : Inport  Port=5
  In6 : Inport  Port=6
  Acceleration : Scope  Commented=on
  Acceleration Computation : MATLAB Function  TreatAsAtomicUnit=on
  Coriolis term : MATLAB Function  TreatAsAtomicUnit=on
  Coriolis term output : Scope  Commented=on
  Damping term : MATLAB Function  TreatAsAtomicUnit=on
  Damping term output : Scope  Commented=on
  Gravitational term output : Scope  Commented=on
  Gravitational terms : MATLAB Function  TreatAsAtomicUnit=on
  Inertial term : Scope  Commented=on
  Integrator : Integrator  InitialCondition=mod_ni_init
  Integrator1 : Integrator  InitialCondition=mod_eta_init
  Kinematic Model : MATLAB Function  TreatAsAtomicUnit=on
  P1 : Subsystem
  P2 : Subsystem
  P3 : Subsystem
  P4 : Subsystem
  P5 : Subsystem
  P6 : Subsystem
  Position and Orientation : Scope  Commented=on
  Relative Velocity : Scope  Commented=on
  Sum : Sum  Inputs=-+--
  Sum1 : Sum  Inputs=|+-
  T output : Scope  Commented=on  NumInputPorts=6
  TAM : MATLAB Function  TreatAsAtomicUnit=on
  TAM output : Scope  Commented=on
  Thruster Velocity Computation : MATLAB Function  TreatAsAtomicUnit=on
  V output : Scope  Commented=on  NumInputPorts=6
  Velocity : Scope  Commented=on
  Velocity in NED : Scope  Commented=on
  seaCurrent Velocity : Scope  Commented=on
  seaCurrent from NED to body : MATLAB Function  TreatAsAtomicUnit=on
  eta : Outport
  ni : Outport  Port=2
  wires:
  P3/1(T3) -> TAM/3(T3), T output/3
  P5/1(T5) -> TAM/5(T5), T output/5
  P6/1(T6) -> TAM/6(T6), T output/6
  Thruster Velocity Computation/6(V6) -> P6/2(V6 [m/s]), V output/6
  Sum/1 -> Acceleration Computation/1(inertialTerm), Inertial term/1
  Integrator/1 -> Kinematic Model/2(ni), Velocity/1, ni/1, Sum1/1  "ni"
  P2/1(T2) -> TAM/2(T2), T output/2
  Acceleration Computation/1(ni_dot) -> Integrator/1, Acceleration/1  "ni_dot"
  Gravitational terms/1(Gterm) -> Sum/1, Gravitational term output/1
  P1/1(T1) -> T output/1, TAM/1(T1)
  TAM/1(tau) -> Sum/2, TAM output/1
  Thruster Velocity Computation/5(V5) -> P5/2(V5 [m/s]), V output/5
  Integrator1/1 -> Position and Orientation/1, Kinematic Model/1(eta), Gravitational terms/1(eta), TAM/7(eta), seaCurrent from NED to body/1(eta), eta/1  "eta"
  Thruster Velocity Computation/2(V2) -> V output/2, P2/2(V2 [m/s])
  Thruster Velocity Computation/1(V1) -> V output/1, P1/2(V1 [m/s])
  Damping term/1(Dterm) -> Damping term output/1, Sum/3
  Kinematic Model/1(eta_dot) -> Integrator1/1, Velocity in NED/1  "eta_dot"
  P4/1(T4) -> TAM/4(T4), T output/4
  Thruster Velocity Computation/4(V4) -> P4/2(V4 [m/s]), V output/4
  Thruster Velocity Computation/3(V3) -> P3/2(V3 [m/s]), V output/3
  Coriolis term/1(Cterm) -> Coriolis term output/1, Sum/4
  In6/1 -> P6/1(n6 [rad/s])
  In2/1 -> P2/1(n2 [rad/s])
  In5/1 -> P5/1(n5 [rad/s])
  In1/1 -> P1/1(n1 [rad/s])
  In4/1 -> P4/1(n4 [rad/s])
  In3/1 -> P3/1(n3 [rad/s])
  seaCurrent from NED to body/1(seaCurrent_Velocity) -> seaCurrent Velocity/1, Sum1/2
  Sum1/1 -> Relative Velocity/1, Thruster Velocity Computation/1(ni_rel), Damping term/1(ni_rel), Coriolis term/1(ni_rel)

== system sim_all/PF/Calcolo distaza pareti ==
  orient : Inport
  pos_es : Inport  Port=2
  Calcolo distanza dalle pareti : MATLAB Function  TreatAsAtomicUnit=on
  Calcolo orientazione dalla parete : MATLAB Function  TreatAsAtomicUnit=on
  dpp : Outport
  dps : Outport  Port=2
  orient_parete : Outport  Port=3
  wires:
  pos_es/1 -> Calcolo distanza dalle pareti/1(pos_es), Calcolo orientazione dalla parete/1(pos_es)
  Calcolo distanza dalle pareti/2(dps) -> dps/1
  Calcolo orientazione dalla parete/1(orient_parete) -> orient_parete/1
  orient/1 -> Calcolo orientazione dalla parete/3(orient)
  Calcolo distanza dalle pareti/1(dpp) -> dpp/1
  [parete_attuale] -> Calcolo distanza dalle pareti/2(parete_attuale), Calcolo orientazione dalla parete/2(parete_attuale)

== system sim_all/PF/Filtro AHRS ==
  AHRS : Inport
  Filtro 1 : DiscreteFir  Coefficients=[0.2 0.2 0.2 0.1 0.1 0.1 0.1]  SampleTime=0.1
  Orientazione : Outport
  wires:
  AHRS/1 -> Filtro 1/1
  Filtro 1/1 -> Orientazione/1

== system sim_all/PF/Filtro DVL ==
  DVL : Inport
  Demux : Demux  Outputs=3
  Filtro 2 : DiscreteFir  Coefficients=[0.3 0.3 0.2 0.2]  SampleTime=0.1
  Filtro 3 : DiscreteFir  Coefficients=[0.3 0.3 0.2 0.2]  SampleTime=0.1
  Mux : Mux  Inputs=3
  Velocità lineare : Outport
  wires:
  Filtro 2/1 -> Mux/1
  Demux/3 -> Mux/3
  DVL/1 -> Demux/1
  Filtro 3/1 -> Mux/2
  Mux/1 -> Velocità lineare/1  "DVL"
  Demux/1 -> Filtro 2/1
  Demux/2 -> Filtro 3/1

== system sim_all/PF/Filtro Gyro ==
  Gyro : Inport
  Filtro 1 : DiscreteFir  Coefficients=[0.9 0.05 0.05]  SampleTime=0.1
  Velocità Angolare : Outport
  wires:
  Gyro/1 -> Filtro 1/1
  Filtro 1/1 -> Velocità Angolare/1

== system sim_all/PF/Gyro_check ==
  Gyro_new : Inport
  MATLAB Function4 : MATLAB Function  TreatAsAtomicUnit=on
  Memory4 : Memory
  flag_Gyro : Outport
  Gyro_now : Outport  Port=2
  wires:
  Gyro_new/1 -> MATLAB Function4/1(gyro_new)
  Memory4/1 -> MATLAB Function4/2(gyro_old)
  MATLAB Function4/1(flag_gyro) -> flag_Gyro/1
  MATLAB Function4/2(gyro_now) -> Memory4/1, Gyro_now/1
